simulink model "RYB_Fault_circuit"  (R2017a)
settings: Solver=VariableStepAuto  StartTime=0.0  StopTime=0.060  MaxStep=1e-4  RelTol=1e-3
libraries: powerlib x8
settings Model: Creator=BHAVESH  LastModifiedBy=BHAVESH

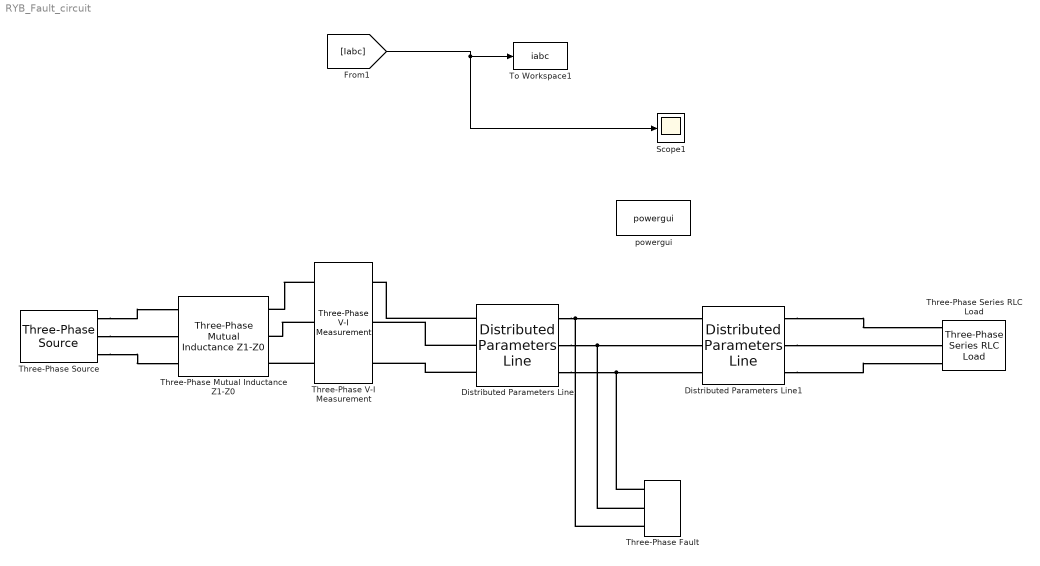
== system RYB_Fault_circuit ==
  Distributed Parameters Line : powerlib/Elements/Distributed Parameters Line  Phases=3  Frequency=50  Resistance=[0.01273 0.3864]  Inductance="[0.9337e-3  4.1264e-3]"  Capacitance=[12.74e-9 7.751e-9]  Length=20  x1=[2.40898090173881e-11 10294.0749186547 10294.0749186547;314.159265358979 314.159265358979 314.159265358979;-2.19695075005325 0.310939601326284 -1.25985672546861]  x2=[2.95209497495067e-11 10223.2477636548 10223.2477636548;314.159265358979 314.159265358979 314.159265358979;-2.30994413421782 0.253079647959442 -1.31771667883545]  x3=[2.79726764763662e-13 64.00818439626 64.0081843962597;314.159265358979 314.159265358979 314.159265358979;2.46552882884176 -2.99037743725855 1.72201154312614]  x4=[1.59129920393986e-13 139.465841648349 139.465841648349;314.159265358979 314.159265358979 314.159265358979;-1.59294874357666 0.216276060158329 -1.35452026663657]  x5=0.000113108313399149  V1=[2.409e-11 1.029e+04 1.029e+04;314.2 314.2 314.2;-2.197 0.3109 -1.26]  V2=[2.952e-11 1.022e+04 1.022e+04;314.2 314.2 314.2;-2.31 0.2531 -1.318]  I1=[2.797e-13 64.01 64.01;314.2 314.2 314.2;2.466 -2.99 1.722]  I2=[1.591e-13 139.5 139.5;314.2 314.2 314.2;-1.593 0.2163 -1.355]  nHarmo=1  Measurements=None
      settings: SourceProductName=Simscape Power Systems
  Distributed Parameters Line1 : powerlib/Elements/Distributed Parameters Line  Phases=3  Frequency=50  Resistance=[0.01273 0.3864]  Inductance="[0.9337e-3  4.1264e-3]"  Capacitance=[12.74e-9 7.751e-9]  Length=20  x1=[2.95489565862825e-11 10223.2477636548 10223.2477636548;314.159265358979 314.159265358979 314.159265358979;-2.29909818683549 0.253079647959442 -1.31771667883545]  x2=[3.95192193152699e-11 10182.2488936876 10182.2488936876;314.159265358979 314.159265358979 314.159265358979;-2.54283129327326 0.194609924330042 -1.37618640246485]  x3=[4.70817270672893e-13 64.0936004777036 64.0936004777035;314.159265358979 314.159265358979 314.159265358979;2.49417307444095 -2.96866427320364 1.74372470718107]  x4=[5.54532918959264e-13 139.359955558189 139.359955558189;314.159265358979 314.159265358979 314.159265358979;-1.45195442182893 0.19460992433004 -1.37618640246485]  x5=0.000113108313399149  V1=[2.955e-11 1.022e+04 1.022e+04;314.2 314.2 314.2;-2.299 0.2531 -1.318]  V2=[3.952e-11 1.018e+04 1.018e+04;314.2 314.2 314.2;-2.543 0.1946 -1.376]  I1=[4.708e-13 64.09 64.09;314.2 314.2 314.2;2.494 -2.969 1.744]  I2=[5.545e-13 139.4 139.4;314.2 314.2 314.2;-1.452 0.1946 -1.376]  nHarmo=1  Measurements=None
      settings: SourceProductName=Simscape Power Systems
  Scope1 : Scope
  Three-Phase Mutual Inductance Z1-Z0 : powerlib/Elements/Three-Phase Mutual Inductance Z1-Z0  LConnTagsString=a|b|c  RConnTagsString=A|B|C  PositiveSequence="[ 2  50e-3]"  ZeroSequence="[4  100e-3]"
      settings: SourceProductName=Simscape Power Systems  SourceProductBaseCode=PS
  Three-Phase Series RLC Load : powerlib/Elements/Three-Phase Series RLC Load  LConnTagsString=A|B|C  Configuration=Y (grounded)  NominalVoltage=1000  Vabc=[1e3 1e3 1e3]  Vabcp=[1e3 1e3 1e3]  NominalFrequency=50  UnbalancedPower=off  ActivePower=10e3  InductivePower=100  CapacitivePower=100  Pabc=[10e3 9e3 11e3]  QLabc=[100 90 110]  QCabc=[100 90 110]  Pabcp=[10e3 9e3 11e3]  QLabcp=[100 90 110]  QCabcp=[100 90 110]  Measurements=None  LoadType=constant Z
  Three-Phase V-I Measurement : powerlib/Measurements/Three-Phase V-I Measurement  VoltageMeasurement=phase-to-ground  SetLabelV=on  LabelV=Vabc  Vpu=off  VpuLL=off  CurrentMeasurement=yes  SetLabelI=on  LabelI=Iabc  Ipu=off  Pbase=100e6  Vbase=500e3  OutputType=Complex  PhasorSimulation=off  PSBequivalent=0
  Three-Phase Fault : powerlib/Elements/Three-Phase Fault  InitialStates=0  FaultA=on  FaultB=on  FaultC=on  GroundFault=on  SwitchTimes="[1/50  5/50]"  External=off  SwitchStatus=NaN  FaultResistance=0.001  GroundResistance=0.10  SnubberResistance=1e6  SnubberCapacitance=inf  Measurements=None
  Three-Phase Source : powerlib/Electrical Sources/Three-Phase Source  InternalConnection=Yg  VoltagePhases=off  Voltage=11e3  PhaseAngle=0  Voltage_phases=[25e3 25e3 25e3]/sqrt(3)  PhaseAngles_phases=[0 -120 +120]  Frequency=50  NonIdealSource=on  SpecifyImpedance=off  Resistance=0.8929  Inductance=16.58e-3  ShortCircuitLevel=100e6  BaseVoltage=11e3  XRratio=7  BusType=swing  Pref=10e3  Qref=0  Prefabc=[10e3, 10e3, 10e3]  Qrefabc=[0, 0, 0]  Qmin=-inf  Qmax=inf
  To Workspace1 : ToWorkspace  VariableName=iabc  SaveFormat=Timeseries  SampleTime=0.001
  powergui : powerlib/powergui  Priority=1  SimulationMode=Continuous  SampleTime=50e-6  frequency=60  Iterations=50  frequencyindice=50  Pbase=100e6  ErrMax=1e-4  UnitsV=kV  UnitsW=MW  buscounter=0  FunctionMessages=off  echomessages=off  EnableUseOfTLC=off  CurrentSourceSwitches=off  DisableSnubberDevices=off  DisableRonSwitches=off  DisableVfSwitches=off  DisplayEquations=off  SolverType=Tustin/Backward Euler (TBE)  Interpol=off  ExternalGateDelay=off  methode=off  Ts=100  x0status=blocks  SPID=on  SwTol=0  HookPort=off  RestoreLinks=warning  ResistiveCurrentMeasurement=off  Frange=[0:2:500]  Ylog=off  Xlog=on  ShowGrid=off  save=off  variable=ZData  structure=0  ZoomFFT=off  StartTime=0.0  cycles=1  DisplayStyle=1  fundamental=60  FreqAxis=off  MaxFrequency=1000  frequencyindicesteady=1  RmsSteady=1  display=off
  wires:
  [Iabc] -> Scope1/1, To Workspace1/1
  connections:
  Distributed Parameters Line/RConn2 -- Three-Phase Fault/LConn2 -- Distributed Parameters Line1/LConn2
  Distributed Parameters Line/RConn3 -- Three-Phase Fault/LConn1 -- Distributed Parameters Line1/LConn3
  Distributed Parameters Line/RConn1 -- Three-Phase Fault/LConn3 -- Distributed Parameters Line1/LConn1
  Three-Phase V-I Measurement/LConn1 -- Three-Phase Mutual Inductance Z1-Z0/RConn1
  Distributed Parameters Line1/RConn1 -- Three-Phase Series RLC Load/LConn1
  Three-Phase V-I Measurement/LConn3 -- Three-Phase Mutual Inductance Z1-Z0/RConn3
  Distributed Parameters Line/LConn3 -- Three-Phase V-I Measurement/RConn3
  Distributed Parameters Line/LConn2 -- Three-Phase V-I Measurement/RConn2
  Distributed Parameters Line1/RConn3 -- Three-Phase Series RLC Load/LConn3
  Distributed Parameters Line1/RConn2 -- Three-Phase Series RLC Load/LConn2
  Three-Phase V-I Measurement/LConn2 -- Three-Phase Mutual Inductance Z1-Z0/RConn2
  Three-Phase Source/RConn2 -- Three-Phase Mutual Inductance Z1-Z0/LConn2
  Distributed Parameters Line/LConn1 -- Three-Phase V-I Measurement/RConn1
  Three-Phase Source/RConn3 -- Three-Phase Mutual Inductance Z1-Z0/LConn3
  Three-Phase Source/RConn1 -- Three-Phase Mutual Inductance Z1-Z0/LConn1
